simulink model "problem2"  (Simulink 7.5)
settings: Solver=ode45  StartTime=0.0  StopTime=20  RelTol=1e-3
settings Model: Creator=philliprivera  LastModifiedBy=philliprivera

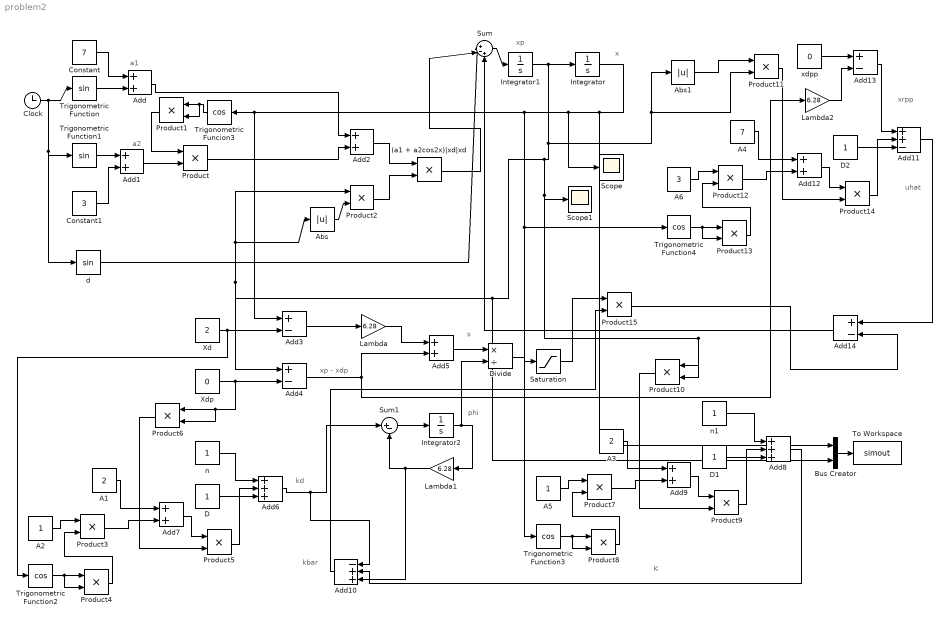
== system problem2 ==
  note: xp
  note: x
  note: a1
  note: a2
  note: s
  note: phi
  note: kd
  note: kbar
  note: K
  note: xp - xdp
  note: xrpp
  note: uhat
  (a1 + a2cos2x)|xd|xd : Product  OutDataType=fixdt(1, 16)  OutScaling=2^0  RndMeth=Zero
  A1 : Constant  Value=2  OutDataType=fixdt(1, 16)  OutScaling=2^0
  A2 : Constant  OutDataType=fixdt(1, 16)  OutScaling=2^0
  A3 : Constant  Value=2  OutDataType=fixdt(1, 16)  OutScaling=2^0
  A4 : Constant  Value=7  OutDataType=fixdt(1, 16)  OutScaling=2^0
  A5 : Constant  OutDataType=fixdt(1, 16)  OutScaling=2^0
  A6 : Constant  Value=3  OutDataType=fixdt(1, 16)  OutScaling=2^0
  Abs : Abs  OutDataType=fixdt(1, 16)  OutScaling=2^0
  Abs1 : Abs  OutDataType=fixdt(1, 16)  OutScaling=2^0
  Add{,1..2,5,7,9,12} (7 alike) : Sum  OutDataType=fixdt(1, 16)  OutScaling=2^-10
  Add10 : Sum  Inputs=-++  OutDataType=fixdt(1, 16)  OutScaling=2^-10
  Add11 : Sum  Inputs=++-  OutDataType=fixdt(1, 16)  OutScaling=2^-10
  Add{3..4,13..14} (4 alike) : Sum  Inputs=+-  OutDataType=fixdt(1, 16)  OutScaling=2^-10
  Add6 : Sum  Inputs=+++  OutDataType=fixdt(1, 16)  OutScaling=2^-10
  Add8 : Sum  Inputs=+++  OutDataType=fixdt(1, 16)  OutScaling=2^-10
  Bus Creator : BusCreator  Inputs=2
  Clock : Clock
      settings: Decimation=10
  Constant : Constant  Value=7  OutDataType=fixdt(1, 16)  OutScaling=2^0
  Constant1 : Constant  Value=3  OutDataType=fixdt(1, 16)  OutScaling=2^0
  D : Constant  OutDataType=fixdt(1, 16)  OutScaling=2^0
  D1 : Constant  OutDataType=fixdt(1, 16)  OutScaling=2^0
  D2 : Constant  OutDataType=fixdt(1, 16)  OutScaling=2^0
  Divide : Product  Inputs=*/  OutDataType=fixdt(1, 16)  OutScaling=2^-10
  Integrator : Integrator  InitialCondition=3
  Integrator1 : Integrator
  Integrator2 : Integrator
  Lambda : Gain  Gain=6.28  ParameterDataType=fixdt(1, 16)  ParameterScaling=2^0  OutDataType=fixdt(1, 16)  OutScaling=2^0
  Lambda1 : Gain  Gain=6.28  ParameterDataType=fixdt(1, 16)  ParameterScaling=2^0  OutDataType=fixdt(1, 16)  OutScaling=2^0
  Lambda2 : Gain  Gain=6.28  ParameterDataType=fixdt(1, 16)  ParameterScaling=2^0  OutDataType=fixdt(1, 16)  OutScaling=2^0
  Product{,1..15} (16 alike) : Product  OutDataType=fixdt(1, 16)  OutScaling=2^0  RndMeth=Zero
  Saturation : Saturate  UpperLimit=1  LowerLimit=-1  OutDataType=fixdt(1, 16)  OutScaling=2^0
  Scope : Scope
      settings: TimeRange=10  YMin=2.5
  Scope1 : Scope
      settings: TimeRange=10  YMin=2.5
  Sum : Sum  Inputs=|+-+  OutDataType=fixdt(1, 16)  OutScaling=2^0
  Sum1 : Sum  Inputs=|+-  OutDataType=fixdt(1, 16)  OutScaling=2^0
  To Workspace : ToWorkspace  VariableName=simout  SampleTime=-1  SaveFormat=Array
  Trigonometric Funcion3 : Trigonometry  Operator=cos
  Trigonometric Function : Trigonometry
  Trigonometric Function1 : Trigonometry
  Trigonometric Function2 : Trigonometry  Operator=cos
  Trigonometric Function3 : Trigonometry  Operator=cos
  Trigonometric Function4 : Trigonometry  Operator=cos
  Xd : Constant  Value=2  OutDataType=fixdt(1, 16)  OutScaling=2^0
  Xdp : Constant  Value=0  OutDataType=fixdt(1, 16)  OutScaling=2^0
  d : Trigonometry
  n : Constant  OutDataType=fixdt(1, 16)  OutScaling=2^0
  n1 : Constant  OutDataType=fixdt(1, 16)  OutScaling=2^0
  xdpp : Constant  Value=0  OutDataType=fixdt(1, 16)  OutScaling=2^0
  wires:
  Clock/1 -> Trigonometric Function/1, Trigonometric Function1/1, d/1
  Constant/1 -> Add/1
  Trigonometric Function/1 -> Add/2
  Constant1/1 -> Add1/2
  Trigonometric Function1/1 -> Add1/1
  Sum/1 -> Integrator1/1
  Integrator/1 -> Trigonometric Function3/1, Trigonometric Function4/1, Trigonometric Funcion3/1, Add3/1, Scope/1, Bus Creator/1
  d/1 -> Sum/1
  Trigonometric Funcion3/1 -> Product1/1, Product1/2
  Product1/1 -> Product/1
  Add1/1 -> Product/2
  Add/1 -> Add2/1
  Product/1 -> Add2/2
  Abs/1 -> Product2/2
  Add2/1 -> (a1 + a2cos2x)|xd|xd/1
  Product2/1 -> (a1 + a2cos2x)|xd|xd/2
  (a1 + a2cos2x)|xd|xd/1 -> Sum/2
  Xd/1 -> Add3/2, Trigonometric Function2/1
  Add3/1 -> Lambda/1
  Xdp/1 -> Add4/2, Product6/1, Product6/2
  Lambda/1 -> Add5/1
  Add4/1 -> Add5/2, Lambda2/1
  Sum1/1 -> Integrator2/1
  Integrator2/1 -> Lambda1/1, Divide/2
  Lambda1/1 -> Sum1/2, Add10/3
  n/1 -> Add6/1
  A1/1 -> Add7/1
  A2/1 -> Product3/1
  Trigonometric Function2/1 -> Product4/1, Product4/2
  Product4/1 -> Product3/2
  Product3/1 -> Add7/2
  Add7/1 -> Product5/1
  Product6/1 -> Product5/2
  Product5/1 -> Add6/2
  D/1 -> Add6/3
  Add6/1 -> Sum1/1, Add10/1
  n1/1 -> Add8/1
  A3/1 -> Add9/1
  A5/1 -> Product7/1
  Trigonometric Function3/1 -> Product8/1, Product8/2
  Product8/1 -> Product7/2
  Product7/1 -> Add9/2
  Add9/1 -> Product9/1
  Product10/1 -> Product9/2
  Product9/1 -> Add8/2
  D1/1 -> Add8/3
  Add8/1 -> Add10/2
  Integrator1/1 -> Integrator/1, Product10/1, Product10/2, Scope1/1, Abs/1, Product2/1, Add4/1, Bus Creator/2, Abs1/1, Product11/2
  A4/1 -> Add12/1
  A6/1 -> Product12/1
  Trigonometric Function4/1 -> Product13/1, Product13/2
  Product13/1 -> Product12/2
  Product12/1 -> Add12/2
  Add12/1 -> Product14/1
  Product11/1 -> Product14/2
  Product14/1 -> Add11/2
  D2/1 -> Add11/3
  Abs1/1 -> Product11/1
  xdpp/1 -> Add13/1
  Lambda2/1 -> Add13/2
  Add13/1 -> Add11/1
  Add11/1 -> Add14/1
  Add5/1 -> Divide/1
  Divide/1 -> Saturation/1
  Saturation/1 -> Product15/1
  Add10/1 -> Product15/2
  Product15/1 -> Add14/2
  Add14/1 -> Sum/3
  Bus Creator/1 -> To Workspace/1
